simulink model "m3"  (R2025a)
settings: Solver=VariableStepAuto  StartTime=0.0  StopTime=0.1  RelTol=1e-3
libraries: spsACVoltageSourceLib x3, spsDetailedThyristorLib x3, spsMultimeterLib x1, spsSeriesRLCBranchLib x1, spspowerguiLib x1
settings Model: Creator=28097  LastModifiedBy=28097

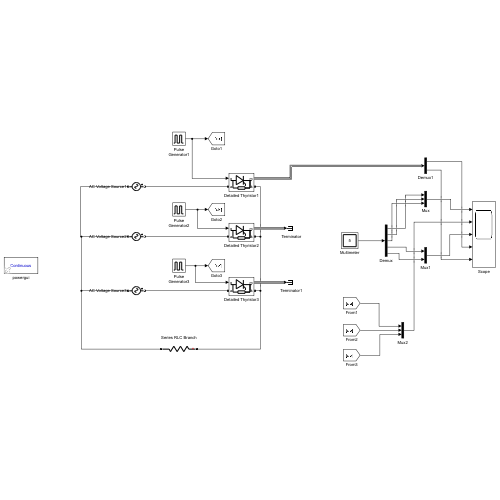
[thumbnail: Simulink's stored preview of the top-level diagram]
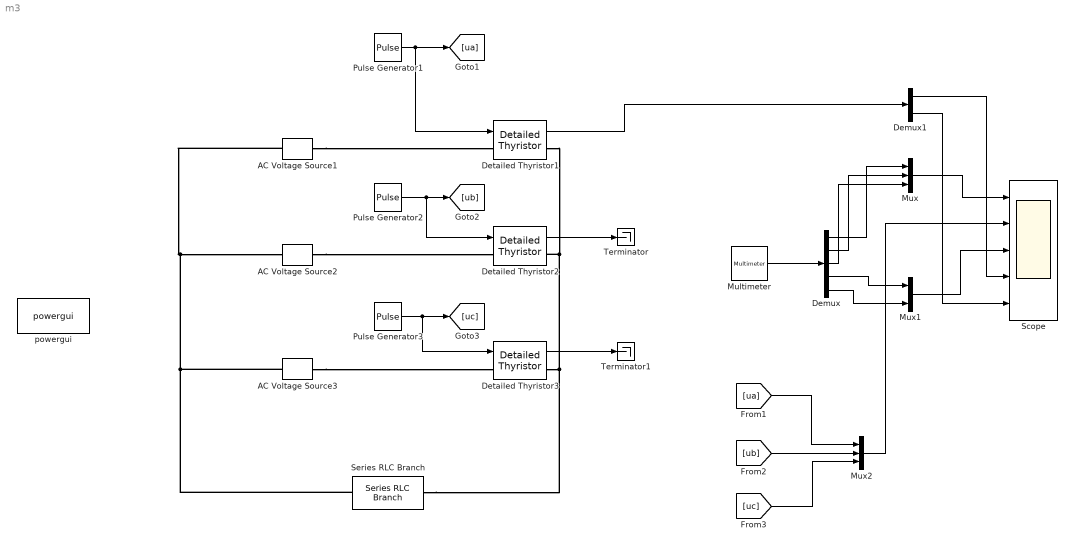
== system m3 ==
  AC Voltage Source1 : spsACVoltageSourceLib/AC Voltage Source  Amplitude=220*sqrt(3)  Phase=0  Frequency=50  SampleTime=0  Measurements=Voltage  BusType=swing  Pref=10e3  Qref=0  Qmin=-inf  Qmax=+inf
  AC Voltage Source2 : spsACVoltageSourceLib/AC Voltage Source  Amplitude=220*sqrt(3)  Phase=-120  Frequency=50  SampleTime=0  Measurements=Voltage  BusType=swing  Pref=10e3  Qref=0  Qmin=-inf  Qmax=+inf
  AC Voltage Source3 : spsACVoltageSourceLib/AC Voltage Source  Amplitude=220*sqrt(3)  Phase=+120  Frequency=50  SampleTime=0  Measurements=Voltage  BusType=swing  Pref=10e3  Qref=0  Qmin=-inf  Qmax=+inf
  Demux : Demux  Outputs=5
  Demux1 : Demux  Outputs=2
  Detailed Thyristor1 : spsDetailedThyristorLib/Detailed Thyristor  Ron=0.001  Lon=1e-3  Vf=0.8  IL=0.1  Tq=100e-6  IC=0  Rs=500  Cs=250e-9  Measurements=on
  Detailed Thyristor2 : spsDetailedThyristorLib/Detailed Thyristor  Ron=0.001  Lon=1e-3  Vf=0.8  IL=0.1  Tq=100e-6  IC=0  Rs=500  Cs=250e-9  Measurements=on
  Detailed Thyristor3 : spsDetailedThyristorLib/Detailed Thyristor  Ron=0.001  Lon=1e-3  Vf=0.8  IL=0.1  Tq=100e-6  IC=0  Rs=500  Cs=250e-9  Measurements=on
  Multimeter : spsMultimeterLib/Multimeter  L=5  sel=[2 3 4 1 5]  Gain=[1 1 1 1 1]  OutputType=Complex  PlotAtSimulationStop=off  PhasorSimulation=off
  Mux : Mux  Inputs=3
  Mux1 : Mux  Inputs=2
  Mux2 : Mux  Inputs=3
  Pulse Generator1 : DiscretePulseGenerator  PulseType=Time based  Amplitude=3  Period=0.02  PulseWidth=5  PhaseDelay=0.02*(30/360)
  Pulse Generator2 : DiscretePulseGenerator  PulseType=Time based  Amplitude=3  Period=0.02  PulseWidth=5  PhaseDelay=0.02*(30/360)+0.02*1/3
  Pulse Generator3 : DiscretePulseGenerator  PulseType=Time based  Amplitude=3  Period=0.02  PulseWidth=5  PhaseDelay=0.02*(30/360)+0.02*2/3
  Scope : Scope  NumInputPorts=5
      settings: ActiveDisplayYMinimum=-475.97159519429897  ActiveDisplayYMaximum=473.23258009716091
  Series RLC Branch : spsSeriesRLCBranchLib/Series RLC Branch  LConnTagsString=__new0  RConnTagsString=__new0  BranchType=R  Resistance=10  Inductance=1e-3  SetiL0=off  InitialCurrent=0  Capacitance=1e-6  Setx0=off  InitialVoltage=0  Measurements=Branch voltage and current
  Terminator : Terminator
  Terminator1 : Terminator
  powergui : spspowerguiLib/powergui  Priority=1  SimulationMode=Continuous  SampleTime=50e-6  frequency=60  Iterations=50  frequencyindice=50  Pbase=100e6  ErrMax=1e-4  UnitsV=kV  UnitsW=MW  buscounter=0  FunctionMessages=off  echomessages=off  EnableUseOfTLC=off  CurrentSourceSwitches=off  DisableSnubberDevices=off  DisableRonSwitches=off  DisableVfSwitches=off  DisplayEquations=off  AutomaticDiscreteSolvers=off  SolverType=Tustin/Backward Euler (TBE)  Interpol=off  ExternalGateDelay=off  methode=off  Ts=100  x0status=blocks  SPID=on  SwTol=0  HookPort=off  NonlinearTolerance=1e-4  nMaxIteration=100  ContinueOnMaxIteration=off  RestoreLinks=warning  ResistiveCurrentMeasurement=off  Frange=[0:2:500]  Ylog=off  Xlog=on  ShowGrid=off  save=off  variable=ZData  structure=0  ZoomFFT=off  StartTime=0.0  cycles=1  DisplayStyle=1  fundamental=60  FreqAxis=off  MaxFrequency=1000  frequencyindicesteady=1  RmsSteady=1  display=off
  wires:
  Pulse Generator1/1 -> Detailed Thyristor1/1, [ua]
  Pulse Generator2/1 -> Detailed Thyristor2/1, [ub]
  Pulse Generator3/1 -> Detailed Thyristor3/1, [uc]
  Detailed Thyristor2/1 -> Terminator/1
  Detailed Thyristor3/1 -> Terminator1/1
  Detailed Thyristor1/1 -> Demux1/1
  [ua] -> Mux2/1
  [ub] -> Mux2/2
  [uc] -> Mux2/3
  Multimeter/1 -> Demux/1
  Demux/1 -> Mux/1
  Demux/2 -> Mux/2
  Demux/3 -> Mux/3
  Demux/4 -> Mux1/1
  Demux/5 -> Mux1/2
  Mux/1 -> Scope/1
  Mux1/1 -> Scope/3
  Demux1/1 -> Scope/4
  Demux1/2 -> Scope/5
  Mux2/1 -> Scope/2
  connections:
  AC Voltage Source1/RConn1 -- Detailed Thyristor1/LConn1
  AC Voltage Source2/RConn1 -- Detailed Thyristor2/LConn1
  AC Voltage Source3/RConn1 -- Detailed Thyristor3/LConn1
  AC Voltage Source1/LConn1 -- Series RLC Branch/RConn1 -- AC Voltage Source3/LConn1 -- AC Voltage Source2/LConn1
  Detailed Thyristor1/RConn1 -- Series RLC Branch/LConn1 -- Detailed Thyristor3/RConn1 -- Detailed Thyristor2/RConn1
